simulink model "Project"  (R2021a)
settings: Solver=ode45  StartTime=0.0  StopTime=5  MaxStep=1e-3  RelTol=1e-3
libraries: spsIGBTDiodeLib x6, simulink x3, spsAsynchronousMachineSIUnitsLib x1, spsDCVoltageSourceLib x1, slpidlib x1, spspowerguiLib x1
settings Model: Creator=Omar  LastModifiedBy=Omar

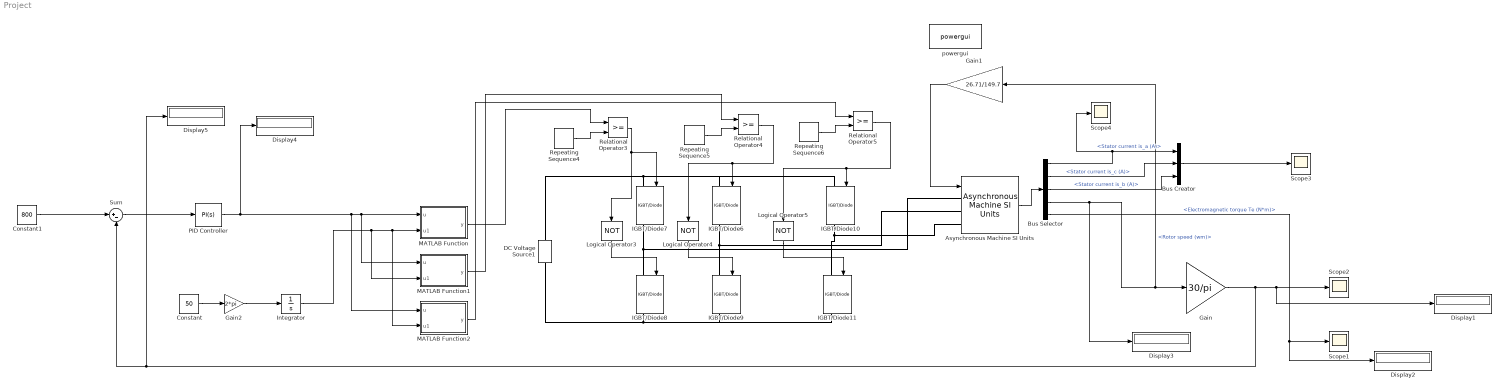
== system Project ==
  Asynchronous Machine SI Units : spsAsynchronousMachineSIUnitsLib/Asynchronous Machine SI Units  RotorType=Squirrel-cage  PresetModel="15:  5.4 HP (4KW)   400 V  50Hz 1430 RPM"  MechanicalLoad=Torque Tm  ShowDetailedParameters=on  ReferenceFrame=Rotor  Units=SI  MeasurementBus=off  NominalParameters=[4000 400 50]  VoltageRatio=1  Stator=[1.405 0.005839]  Rotor=[1.395 0.005839]  Cage1=[0.4155 0.002066]  Cage2=[0.4168 0.0003495]  Lm=0.1722  Mechanical=[0.0131 0.002985 2]  PolePairs=2  InitialConditions=[1 0 0 0 0 0 0 0]  SimulateSaturation=off  Saturation=[14.03593122, 27.81365428, 53.79336849, 72.68890987, 97.98006896, 148.6815601, 215.7428561, 302.9841135, 428.7778367 ; 230, 322, 414, 460, 506, 552, 598, 644, 690]  LoadFlowParameters=1492000  TsPowergui=0  TsBlock=-1  IterativeModel=Trapezoidal non iterative  IterativeDiscreteModel=Trapezoidal non iterative  Pmec=1.492e+006
  Bus Creator : BusCreator  Inputs=3
  Bus Selector : BusSelector  OutputSignals=Stator measurements.Stator current is_a (A),Stator measurements.Stator current is_c (A),Stator measurements.Stator current is_b (A),Mechanical.Rotor speed (wm),Mechanical.Electromagnetic torque Te (N*m)
  Constant : Constant  Value=50
  Constant1 : Constant  Value=800
  DC Voltage Source1 : spsDCVoltageSourceLib/DC Voltage Source  Amplitude=666.53  Measurements=None
  Display{1..5} (5 alike) : Display
  Gain : Gain  Gain=30/pi
  Gain1 : Gain  Gain=26.71/149.7
  Gain2 : Gain  Gain=2*pi
  IGBT/Diode{6..11} (6 alike) : spsIGBTDiodeLib/IGBT//Diode  Ron=1e-3  Rs=1e5  Cs=inf  Measurements=on
  Integrator : Integrator
  Logical Operator3 : Logic  Operator=NOT  AllPortsSameDT=off  OutDataTypeStr=boolean
  Logical Operator4 : Logic  Operator=NOT  AllPortsSameDT=off  OutDataTypeStr=boolean
  Logical Operator5 : Logic  Operator=NOT  AllPortsSameDT=off  OutDataTypeStr=boolean
  MATLAB Function : MATLAB Function  TreatAsAtomicUnit=on
  MATLAB Function1 : MATLAB Function  TreatAsAtomicUnit=on
  MATLAB Function2 : MATLAB Function  TreatAsAtomicUnit=on
  PID Controller : slpidlib/PID Controller  Controller=PI  Form=Parallel  TimeDomain=Continuous-time  UseExternalTs=off  SampleTime=-1  IntegratorMethod=Forward Euler  FilterMethod=Forward Euler  ControllerParametersSource=internal  P=0.0001  I=0.008  D=0.1  UseFilter=on  N=100  TunerSelectOption=Frequency Response Based  InitialConditionSource=internal  InitialConditionForIntegrator=0  InitialConditionForFilter=0  DifferentiatorICPrevScaledInput=0  ExternalReset=none  TrackingMode=off  Kt=1  LimitOutput=on  SatLimitsSource=internal  UpperSaturationLimit=0.98  LowerSaturationLimit=-0.98  LinearizeAsGain=on  AntiWindupMode=clamping  Kb=1  POutMin=[]  POutMax=[]  IOutMin=[]  IOutMax=[]  DOutMin=[]  DOutMax=[]  NOutMin=[]  NOutMax=[]  SumOutMin=[]  SumOutMax=[]  SaturationOutMin=[]  SaturationOutMax=[]  PParamMin=[]  PParamMax=[]  IParamMin=[]  IParamMax=[]  DParamMin=[]  DParamMax=[]  NParamMin=[]  NParamMax=[]  KbParamMin=[]  KbParamMax=[]  KtParamMin=[]  KtParamMax=[]  KbOutMin=[]  KbOutMax=[]  KtOutMin=[]  KtOutMax=[]  IntegratorOutMin=[]  IntegratorOutMax=[]  FilterOutMin=[]  FilterOutMax=[]  SumI1OutMin=[]  SumI1OutMax=[]  SumI2OutMin=[]  SumI2OutMax=[]  SumI3OutMin=[]  SumI3OutMax=[]  SumI4OutMin=[]  SumI4OutMax=[]  SumDOutMin=[]  SumDOutMax=[]  DifferentiatorOutMin=[]  DifferentiatorOutMax=[]  FilterDiffOutCoefMin=[]  FilterDiffOutCoefMax=[]  ReciprocalOutMin=[]  ReciprocalOutMax=[]  SumDenOutMin=[]  SumDenOutMax=[]  SumNumOutMin=[]  SumNumOutMax=[]  DivideOutMin=[]  DivideOutMax=[]  UdiffTsProdOutMin=[]  UdiffTsProdOutMax=[]  NTsProdOutMin=[]  NTsProdOutMax=[]  UintegralTsProdOutMin=[]  UintegralTsProdOutMax=[]  UngainTsProdOutMin=[]  UngainTsProdOutMax=[]  IntegratorContinuousStateAttributes=''  IntegratorStateMustResolveToSignalObject=off  IntegratorRTWStateStorageClass=Auto  FilterContinuousStateAttributes=''  FilterStateMustResolveToSignalObject=off  FilterRTWStateStorageClass=Auto  ParallelPVariant=InternalParameters  IdealPVariant=Disabled  IVariant=InternalParameters  DVariant=Disabled  IntegratorVariant=Continuous  SatVariant=Enabled  AWVariant=ContClampingParallel  PCopyVariant=Disabled  TRVariant=Disabled  FdbkBlocksVariant=Forward  IdealPFdbkVariant=Disabled  SatFdbkVariant=Disabled  DerivativeFilterVariant=Disabled  NVariant=Disabled  NCopyVariant=Disabled_SignalSpec  FilterICVariant=Disabled  IntegratorICVariant=InternalICs  ExternalResetVariant=Disabled  TRSumVariant=Passthrough  SumFdbkVariant=Disabled  SumVariant=Sum_PI  TsampFilterVariant=InternalTs  TsampNgainVariant=Passthrough  TsampIntegralVariant=Passthrough  ExternalSaturationOutDataTypeStr=Inherit: Same as second input
  Relational Operator3 : RelationalOperator  OutDataTypeStr=boolean  RndMeth=Simplest
  Relational Operator4 : RelationalOperator  OutDataTypeStr=boolean  RndMeth=Simplest
  Relational Operator5 : RelationalOperator  OutDataTypeStr=boolean  RndMeth=Simplest
  Repeating Sequence4 : simulink/Sources/Repeating Sequence  rep_seq_t=[0 (1/5050)/4 (1/5050)/2 (3/5050)/4 (1/5050) ]  rep_seq_y=[0 1 0 -1 0]
  Repeating Sequence5 : simulink/Sources/Repeating Sequence  rep_seq_t=[0 (1/5050)/4 (1/5050)/2 (3/5050)/4 (1/5050) ]  rep_seq_y=[0 1 0 -1 0]
  Repeating Sequence6 : simulink/Sources/Repeating Sequence  rep_seq_t=[0 (1/5050)/4 (1/5050)/2 (3/5050)/4 (1/5050) ]  rep_seq_y=[0 1 0 -1 0]
  Scope{1..4} (4 alike) : Scope
  Sum : Sum  Inputs=|+-
  powergui : spspowerguiLib/powergui  Priority=1  SimulationMode=Discrete  SampleTime=1e-6  frequency=60  Iterations=50  frequencyindice=0  Pbase=100e6  ErrMax=1e-4  UnitsV=kV  UnitsW=MW  buscounter=0  FunctionMessages=off  echomessages=off  EnableUseOfTLC=off  CurrentSourceSwitches=off  DisableSnubberDevices=off  DisableRonSwitches=off  DisableVfSwitches=off  DisplayEquations=off  AutomaticDiscreteSolvers=off  SolverType=Tustin/Backward Euler (TBE)  Interpol=off  ExternalGateDelay=off  methode=off  Ts=100  x0status=blocks  SPID=on  SwTol=0  HookPort=off  NonlinearTolerance=1e-4  nMaxIteration=100  ContinueOnMaxIteration=off  RestoreLinks=warning  ResistiveCurrentMeasurement=off  Frange=[0:2:500]  Ylog=off  Xlog=on  ShowGrid=off  save=off  variable=ZData  structure=0  ZoomFFT=off  StartTime=0.0  cycles=1  DisplayStyle=1  fundamental=60  FreqAxis=off  MaxFrequency=1000  frequencyindicesteady=1  RmsSteady=1  display=off
  wires:
  Gain/1 -> Display5/1, Sum/2, Display1/1, Scope2/1
  Asynchronous Machine SI Units/1 -> Bus Selector/1
  Bus Selector/4 -> Display3/1, Gain1/1, Gain/1  "<Rotor speed (wm)>"
  Bus Selector/5 -> Display2/1, Scope1/1  "<Electromagnetic torque Te (N*m)>"
  Bus Selector/1 -> Bus Creator/1, Scope4/1  "<Stator current is_a (A)>"
  Bus Selector/2 -> Bus Creator/2  "<Stator current is_c (A)>"
  Bus Selector/3 -> Bus Creator/3  "<Stator current is_b (A)>"
  Bus Creator/1 -> Scope3/1
  Gain1/1 -> Asynchronous Machine SI Units/1
  Gain2/1 -> Integrator/1
  Integrator/1 -> MATLAB Function1/2(u1), MATLAB Function2/2(u1), MATLAB Function/2(u1)
  MATLAB Function/1(y) -> Relational Operator3/1
  Logical Operator5/1 -> IGBT/Diode11/1
  Logical Operator3/1 -> IGBT/Diode8/1
  MATLAB Function1/1(y) -> Relational Operator4/1
  Repeating Sequence5/1 -> Relational Operator4/2
  Repeating Sequence4/1 -> Relational Operator3/2
  Relational Operator3/1 -> IGBT/Diode7/1, Logical Operator3/1
  Relational Operator5/1 -> IGBT/Diode10/1, Logical Operator5/1
  Relational Operator4/1 -> IGBT/Diode6/1, Logical Operator4/1
  Repeating Sequence6/1 -> Relational Operator5/2
  MATLAB Function2/1(y) -> Relational Operator5/1
  Logical Operator4/1 -> IGBT/Diode9/1
  Sum/1 -> PID Controller/1
  Constant1/1 -> Sum/1
  PID Controller/1 -> MATLAB Function2/1(u), MATLAB Function1/1(u), MATLAB Function/1(u), Display4/1
  Constant/1 -> Gain2/1
  connections:
  IGBT/Diode8/RConn1 -- IGBT/Diode11/RConn1 -- IGBT/Diode9/RConn1 -- DC Voltage Source1/LConn1
  IGBT/Diode7/LConn1 -- IGBT/Diode10/LConn1 -- IGBT/Diode6/LConn1 -- DC Voltage Source1/RConn1
  IGBT/Diode10/RConn1 -- IGBT/Diode11/LConn1 -- Asynchronous Machine SI Units/LConn3
  IGBT/Diode7/RConn1 -- Asynchronous Machine SI Units/LConn1 -- IGBT/Diode8/LConn1
  IGBT/Diode6/RConn1 -- Asynchronous Machine SI Units/LConn2 -- IGBT/Diode9/LConn1

== matlab function Project/MATLAB Function ==
  data: u input; y output; u1 input
function y = fcn(u , u1)

y = u*sin(u1);

== matlab function Project/MATLAB Function2 ==
  data: u input; y output; u1 input
function y = fcn(u , u1)

y = u*sin(u1 + ((2*pi)/3));

== matlab function Project/MATLAB Function1 ==
  data: u input; y output; u1 input
function y = fcn(u ,u1)

y = u*sin(u1 - ((2*pi)/3));
